simulink library "World_Config_Utilities"  (R2022a)
settings: Solver=VariableStepAuto  StartTime=0.0  StopTime=10.0  RelTol=1e-3
undefined symbols (not defined in the file or in its folder): acc_theta, accel_ramp_rate, hp_rc_wld_t, qt, time_vector, xyz_matrix
libraries: sm_lib x6, nesl_utility x5, simulink x1, Scene_Systems x1, $bdroot x1
Description:
  | Simscape Vehicle Templates Library
  | 
  | Copyright 2018-2024 The MathWorks, Inc.
settings Model: Creator=smiller  LastModifiedBy=smiller

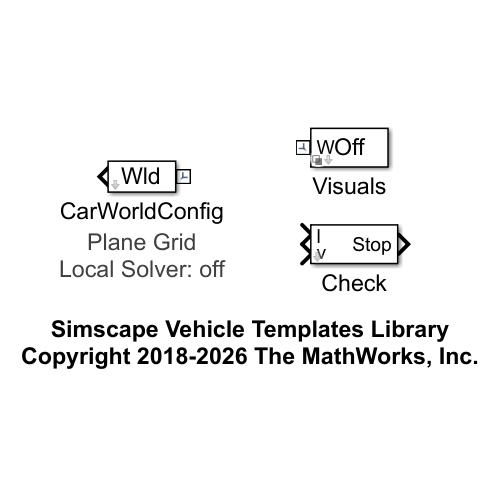
[thumbnail: Simulink's stored preview of the top-level diagram]
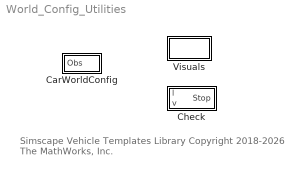
== system World_Config_Utilities ==
  note: Simscape Vehicle Templates Library
      | Copyright 2018-2026 The MathWorks, Inc.
  CarWorldConfig : Subsystem  mask(Environment){UseLocalSolver=off, LocalSolverChoice=Backward Euler, LocalSolverSampleTime=0.005, DoFixedCost=off, MaxNonlinIter=3, popup_scene=Plane Grid, popup_gravity=Constant, GravityVector=[0 0 -9.80665], popup_vis_point=Off, time_vector=qt, xyz_matrix=hp_rc_wld_t, clr_vis=[0.0 1.0 0.8], opc_vis=0.6, rad_vis=0.03}
      mask prompts: UseLocalSolver "Use Local Solver"; LocalSolverChoice "Solver Type:"; LocalSolverSampleTime "Sample time"; DoFixedCost "Use fixed-cost"; MaxNonlinIter "Number of iterations"; popup_scene "Scene"; popup_gravity "Gravity Model"; GravityVector "Gravity Vector [x y z] (m/s^2)"; popup_vis_point "Visualize Point"; time_vector "Time Vector [nx1] (sec)"; xyz_matrix "Coordinates [nx3] (m)"; clr_vis "Color [R G B] (0-1)"; opc_vis "Opacity (0-1)"; rad_vis "Radius (m)"
      mask help: World frame, driving surface, gravity, and solver settings.
      mask init:
      | if(LocalSolverChoice == 1)
      |     solverChoice = 'NE_BACKWARD_EULER_ADVANCER';
      | elseif(LocalSolverChoice == 2)
      |     solverChoice = 'NE_TRAPEZOIDAL_ADVANCER';
      | elseif(LocalSolverChoice == 3)
      |     solverChoice = 'NE_PARTITIONING_ADVANCER';
      | end
      | set_param([gcb '/Solver Configuration'],'LocalSolverChoice',solverChoice)
      | 
      | tempblkscenename = strrep(get_param(gcb,'popup_scene'),' ','_');
      | set_param([gcb '/Scene'],'LabelModeActiveChoice',tempblkscenename);
      | gravityModel = get_param(gcb,'popup_gravity');
      | if(strcmpi(gravityModel,'constant'))
      |     set_param([gcb '/Mechanism Configuration'],'LabelModeActiveChoice','ConstantGravity');
      | elseif(strcmpi(gravityModel,'ramp x and y components'))
      |     set_param([gcb '/Mechanism Configuration'],'LabelModeActiveChoice','VariableGravityXY');
      | end
      | clear tempblkscenename
      settings: AttributesFormatString=|
      | %<popup_scene>
      | Local Solver: %<UseLocalSolver>
      mask TypeOptions UseLocalSolver:
      | Solver
      | Configuration/UseLocalSolver
      mask Callback UseLocalSolver:
      | maskObj = Simulink.Mask.get(gcb);
      | 
      | samTM_h = maskObj.getParameter('LocalSolverSampleTime');
      | slvCH_h = maskObj.getParameter('LocalSolverChoice');
      | fixCT_h = maskObj.getParameter('DoFixedCost');
      | 
      | temp_useLSstate = get_param(gcb,'UseLocalSolver');
      | samTM_h.Enabled = temp_useLSstate;
      | slvCH_h.Enabled = temp_useLSstate;
      | fixCT_h.Enabled = temp_useLSstate;
      | 
      | clear maskObj
      | clear samTM_h slvCH_h fixCT_h
      | clear temp_useLSstate
      mask TypeOptions LocalSolverChoice: Backward Euler | Trapezoidal Rule | Partitioning
      mask TypeOptions LocalSolverSampleTime:
      | Solver
      | Configuration/LocalSolverSampleTime
      mask TypeOptions DoFixedCost:
      | Solver
      | Configuration/DoFixedCost
      mask Callback DoFixedCost:
      | maskObj = Simulink.Mask.get(gcb);
      | 
      | numIT_h = maskObj.getParameter('MaxNonlinIter');
      | 
      | temp_doFixCoststate = get_param(gcb,'DoFixedCost');
      | numIT_h.Enabled = temp_doFixCoststate;
      | 
      | clear maskObj numIT_h temp_doFixCoststate
      mask TypeOptions MaxNonlinIter:
      | Solver
      | Configuration/MaxNonlinIter
      mask TypeOptions popup_scene: Plane Grid | Road Two Lane | Double Lane Change | Double Lane Change ISO3888 | Slalom | Ice Patch | Elk Test | RDF Rough Road | Rough Road Z Only | CRG Rough Road | RDF Plateau | Plateau Z Only | CRG Plateau | Track Mallory Park | Track Mallory Park Obstacle | MCity | CRG Hockenheim | CRG Hockenheim F | CRG Kyalami | CRG Kyalami F | CRG Mallory Park | CRG Mallory Park F | CRG Nurburgring N | CRG Nurburgring N F | CRG Pikes Peak | CRG Suzuka | CRG Suzuka F | CRG Custom | CRG Custom F | GS Uneven Road | GS Grid Surface | Skidpad | Constant Radius | Testrig 4 Post
      mask TypeOptions popup_gravity: Constant | Ramp x and y components
      mask TypeOptions popup_vis_point: Visuals/popup_vis_point
      mask Callback popup_vis_point:
      | bh = gcb;
      | maskObj = Simulink.Mask.get(bh); % Get the mask object of the current block
      | tvec_h  = maskObj.getParameter('time_vector'); % Get the parameter to hide
      | xyz_h   = maskObj.getParameter('xyz_matrix'); % Get the parameter to hide
      | 
      | clr_h   = maskObj.getParameter('clr_vis'); % Get the parameter to hide
      | opc_h   = maskObj.getParameter('opc_vis'); % Get the parameter to hide
      | rad_h   = maskObj.getParameter('rad_vis'); % Get the parameter to hide
      | 
      | % Check the value of ControlParam
      | enaVisPnt = get_param(bh, 'popup_vis_point');
      | 
      | tvec_h.Visible  = 'off';
      | xyz_h.Visible  = 'off';
      | clr_h.Visible  = 'off';
      | opc_h.Visible  = 'off';
      | rad_h.Visible  = 'off';
      | 
      | if strcmp(enaVisPnt, 'On')
      |     tvec_h.Visible  = 'on';
      |     xyz_h.Visible   = 'on';
      |     clr_h.Visible   = 'on';
      |     opc_h.Visible   = 'on';
      |     rad_h.Visible   = 'on';
      | end
      mask TypeOptions time_vector: Visuals/time_vector
      mask TypeOptions xyz_matrix: Visuals/xyz_matrix
      mask TypeOptions clr_vis: Visuals/clr_vis
      mask TypeOptions opc_vis: Visuals/opc_vis
      mask TypeOptions rad_vis: Visuals/rad_vis
      mask Display: disp('Wld')
  Check : Subsystem  mask(Stop Conditions){stop_speed=0.1, start_check_time=5, max_speed=0.4, start_check_time_max_speed=20000, lat_dev_threshold=8, start_check_time_ld=10000, end_lap_num=1, start_check_time_end_lap=10000, max_dist_threshold=10000, start_check_time_max_dist=10000}
      mask help: Check conditions of vehicle to determine if simulation should stop. Conditions can include speed, position, or end of lap. Set time to start check to very high values to prevent condition from stopping simulation.
      mask TypeOptions stop_speed: Stop Threshold/Value
      mask TypeOptions start_check_time: Start Checking/Time
      mask TypeOptions max_speed: Max Speed Threshold/Value
      mask TypeOptions start_check_time_max_speed: Start Checking Max Speed/Time
      mask TypeOptions lat_dev_threshold: Lateral Deviation Threshold/Value
      mask TypeOptions start_check_time_ld: Start Checking Lat Dev/Time
      mask TypeOptions end_lap_num: End Lap/Value
      mask TypeOptions start_check_time_end_lap: Start Checking End Lap/Time
      mask TypeOptions max_dist_threshold: End Distance/Value
      mask TypeOptions start_check_time_max_dist: Start Checking End Distance/Time
      mask DialogControl text_quantity Prompt: Quantity
      mask DialogControl text_start_check Prompt: Start Check (sec)
      mask DialogControl text_final_speed Prompt: Final Speed (m/s)
      mask DialogControl text_max_speed Prompt: Max Speed (m/s)
      mask DialogControl text_max_lat_dev Prompt: Max Lateral Offset (m)
      mask DialogControl text_end_lap_1 Prompt: End Lap
      mask DialogControl text_max_distance Prompt: Max Distance
  Visuals : Subsystem  Variant=on  VariantControlMode=label  VariantControl=Choice  LabelModeActiveChoice=Off  mask{popup_vis_point=Off, time_vector=time_vector, xyz_matrix=xyz_matrix, clr_vis=[0.0 1.0 0.8], opc_vis=0.6, rad_vis=0.03}
      mask prompts: popup_vis_point "Visualize Point"; time_vector "Time Vector [nx1] (sec)"; xyz_matrix "Coordinates [nx3] (m)"; clr_vis "Color [R G B] (0-1)"; opc_vis "Opacity (0-1)"; rad_vis "Radius (m)"
      mask init:
      | bh = gcb;
      | pvisPt = get_param(bh,'popup_vis_point');
      | if(strcmp(pvisPt,'Off'))
      |     time_vector = [0];
      |     xyz_matrix =  [0 0 0];
      | end
      | set_param(bh,'LabelModeActiveChoice',pvisPt)
      mask TypeOptions popup_vis_point: Off | On
      mask Callback popup_vis_point:
      | bh = gcb;
      | maskObj = Simulink.Mask.get(bh); % Get the mask object of the current block
      | tvec_h  = maskObj.getParameter('time_vector'); % Get the parameter to hide
      | xyz_h   = maskObj.getParameter('xyz_matrix'); % Get the parameter to hide
      | clr_h   = maskObj.getParameter('clr_vis'); % Get the parameter to hide
      | opc_h   = maskObj.getParameter('opc_vis'); % Get the parameter to hide
      | rad_h   = maskObj.getParameter('rad_vis'); % Get the parameter to hide
      | 
      | % Check the value of ControlParam
      | enaVisPnt = get_param(bh, 'popup_vis_point');
      | 
      | tvec_h.Visible  = 'off';
      | xyz_h.Visible  = 'off';
      | clr_h.Visible  = 'off';
      | opc_h.Visible  = 'off';
      | rad_h.Visible  = 'off';
      | 
      | if strcmp(enaVisPnt, 'On')
      |     tvec_h.Visible  = 'on';
      |     xyz_h.Visible   = 'on';
      |     clr_h.Visible   = 'on';
      |     opc_h.Visible   = 'on';
      |     rad_h.Visible   = 'on';
      | end

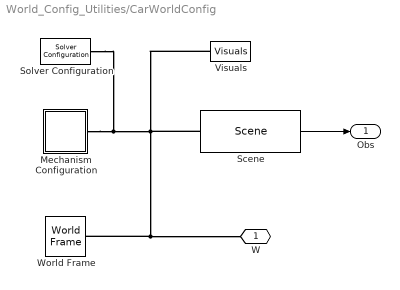
== system World_Config_Utilities/CarWorldConfig ==
  Mechanism Configuration : Subsystem  Variant=on  VariantControlMode=label  VariantControl=Choice  LabelModeActiveChoice=ConstantGravity
      settings: AttributesFormatString=%<LabelModeActiveChoice>
      mask Display: disp(' ');
  Scene : Scene_Systems/Scene  SystemSampleTime=-1  LabelModeActiveChoice=Plane_Grid  VariantActivationTime=update diagram  Latency=0  AutoFrameSizeCalculation=off
      settings: AttributesFormatString=%<LabelModeActiveChoice>
  Solver Configuration : nesl_utility/Solver Configuration  PhysicalDomain=network_engine_domain  SubClassName=solver  LeftPortType=input  RightPortType=generic  Tones=[]  Harmonics=[]  SimulateNoise=off  Profile=off  UseLocalSampling=off  EnableSwitchedLinearOptims=on  FrequencyDomain=off  UseCCode=off  RelTol=0.001  AbsTol=1e-06  MinStep=1e-09  ToWorkspace=off  RevertToSquareIcSolve=off  NumHomotopyIterations=100  PhasorMode=off  PhasorModeNumHarmonics=1  IndexReductionMethod=DerivativeReplacement  DoDC=off  ResidualTolerance=1e-9  UseLocalSolver=off  LocalSolverChoice=NE_BACKWARD_EULER_ADVANCER  LocalSolverSampleTime=LocalSolverSampleTime  DoFixedCost=off  MaxNonlinIter=MaxNonlinIter  MaxModeIter=2  ComputeImpulses=off  ImpulseIterations=2  LinearAlgebra=Sparse  LinearAlgebraNumThread=0  EquationFormulation=NE_TIME_EF  DelaysMemoryBudget=1024  AutomaticFiltering=on  FilteringTimeConstant=0.001  PartitionStorageMethod=AS_NEEDED  PartitionMemoryBudget=1024  PartitionMethod=FAST
      settings: SourceProductBaseCode=SS,PW,VE
  Visuals : $bdroot/Visuals  VariantControl=Choice  LabelModeActiveChoice=Off  popup_vis_point=Off  time_vector=time_vector  xyz_matrix=xyz_matrix  clr_vis=clr_vis  opc_vis=opc_vis  rad_vis=rad_vis
  World Frame : sm_lib/Frames and Transforms/World Frame
  W : PMIOPort  Side=Left
  Obs : Outport  VectorParamsAs1DForOutWhenUnconnected=off
  wires:
  Scene/1 -> Obs/1
  connections:
  Solver Configuration/RConn1 -- Mechanism Configuration/RConn1 -- Visuals/LConn1 -- World Frame/RConn1 -- W/RConn1 -- Scene/LConn1

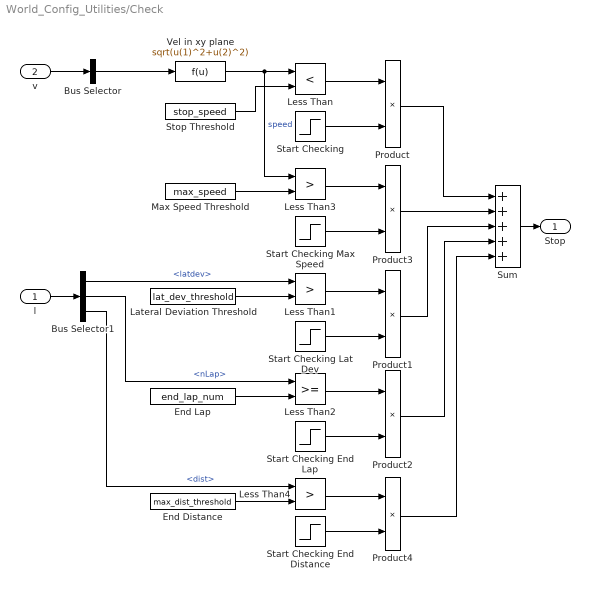
== system World_Config_Utilities/Check ==
  l : Inport
  v : Inport  Port=2
  Bus Selector : BusSelector  OutputSignals=World.vx,World.vy  OutputAsBus=on
  Bus Selector1 : BusSelector  OutputSignals=Reference.latdev,Reference.nLap,Reference.dist
  End Distance : Constant  Value=max_dist_threshold
  End Lap : Constant  Value=end_lap_num
  Lateral Deviation Threshold : Constant  Value=lat_dev_threshold
  Less Than : RelationalOperator  Operator=<  OutDataTypeStr=boolean  RndMeth=Simplest  InputSameDT=off
  Less Than1 : RelationalOperator  Operator=>  OutDataTypeStr=boolean  ZeroCross=off  RndMeth=Simplest  InputSameDT=off
  Less Than2 : RelationalOperator  OutDataTypeStr=boolean  RndMeth=Simplest  InputSameDT=off
  Less Than3 : RelationalOperator  Operator=>  OutDataTypeStr=boolean  RndMeth=Simplest  InputSameDT=off
  Less Than4 : RelationalOperator  Operator=>  OutDataTypeStr=boolean  ZeroCross=off  RndMeth=Simplest  InputSameDT=off
  Max Speed Threshold : Constant  Value=max_speed
  Product{,1..4} (5 alike) : Product
  Start Checking : Step  Time=start_check_time  SampleTime=0  ZeroCross=off
  Start Checking End Distance : Step  Time=start_check_time_max_dist  SampleTime=0  ZeroCross=off
  Start Checking End Lap : Step  Time=start_check_time_end_lap  SampleTime=0  ZeroCross=off
  Start Checking Lat Dev : Step  Time=start_check_time_ld  SampleTime=0  ZeroCross=off
  Start Checking Max Speed : Step  Time=start_check_time_max_speed  SampleTime=0  ZeroCross=off
  Stop Threshold : Constant  Value=stop_speed
  Sum : Sum  Inputs=+++++
  Vel in xy plane : Fcn  Expr=sqrt(u(1)^2+u(2)^2)
  Stop : Outport  VectorParamsAs1DForOutWhenUnconnected=off
  wires:
  Bus Selector1/2 -> Less Than2/1  "<nLap>"
  Product3/1 -> Sum/2
  Max Speed Threshold/1 -> Less Than3/2
  Less Than3/1 -> Product3/1
  Start Checking Max Speed/1 -> Product3/2
  Product2/1 -> Sum/4
  Start Checking End Lap/1 -> Product2/2
  Less Than2/1 -> Product2/1
  End Lap/1 -> Less Than2/2
  Product1/1 -> Sum/3
  Sum/1 -> Stop/1
  Start Checking Lat Dev/1 -> Product1/2
  Less Than1/1 -> Product1/1
  Lateral Deviation Threshold/1 -> Less Than1/2
  Bus Selector1/1 -> Less Than1/1  "<latdev>"
  l/1 -> Bus Selector1/1
  Vel in xy plane/1 -> Less Than3/1, Less Than/1  "speed"
  Bus Selector/1 -> Vel in xy plane/1
  Product/1 -> Sum/1
  Start Checking/1 -> Product/2
  v/1 -> Bus Selector/1
  Stop Threshold/1 -> Less Than/2
  Less Than/1 -> Product/1
  End Distance/1 -> Less Than4/2
  Bus Selector1/3 -> Less Than4/1  "<dist>"
  Less Than4/1 -> Product4/1
  Start Checking End Distance/1 -> Product4/2
  Product4/1 -> Sum/5

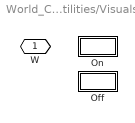
== system World_Config_Utilities/Visuals ==
  Off : Subsystem  VariantControl=Off
  On : Subsystem  VariantControl=On  mask{tvec=time_vector, visp1=xyz_matrix, clr_vis=clr_vis, opc_vis=opc_vis, rad_vis=rad_vis}
      mask prompts: tvec "Time Vector (s)"; visp1 "Coordinates [x y z] (s)"; clr_vis "Color [R G B] (0-1)"; opc_vis "Opacity (0-1)"; rad_vis "Radius (m)"
      mask init:
      | % Ensure matrices have correct dimensions
      | if(size(tvec,2)>1)
      |     t_vec = tvec';
      | else
      |     t_vec = tvec;
      | end
      | 
      | if(size(visp1,2)>3)
      |     vis_p1 = visp1';
      | else
      |     vis_p1 = visp1;
      | end
      | 
      | if((size(t_vec,1)==size(vis_p1,1)) && ...
      |         size(vis_p1,2)==3)
      | else
      |     % If not valid set of data, leave vis at [0 0 0]
      |     % and warn user.
      |     t_vec = 0;
      |     vis_p1 = [0 0 0];
      |     warning('Visualization data not defined correctly.')
      | end
  W : PMIOPort  Side=Left

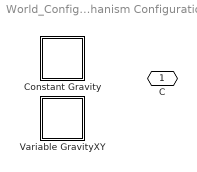
== system World_Config_Utilities/CarWorldConfig/Mechanism Configuration ==
  Constant Gravity : Subsystem  VariantControl=ConstantGravity
  Variable GravityXY : Subsystem  VariantControl=VariableGravityXY
  C : PMIOPort  Side=Right

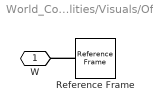
== system World_Config_Utilities/Visuals/Off ==
  Reference Frame : sm_lib/Frames and Transforms/Reference Frame
  W : PMIOPort  Side=Left
  connections:
  Reference Frame/RConn1 -- W/RConn1

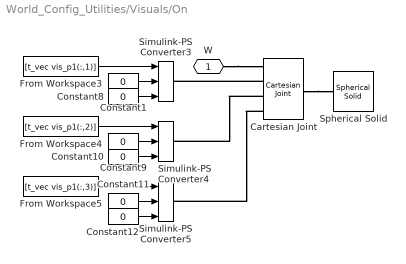
== system World_Config_Utilities/Visuals/On ==
  Cartesian Joint : sm_lib/Joints/Cartesian Joint  JointMode=Normal  SenseConstraintForce=off  SenseConstraintForceX=off  SenseConstraintForceY=off  SenseConstraintForceZ=off  SenseConstraintTorque=off  SenseConstraintTorqueX=off  SenseConstraintTorqueY=off  SenseConstraintTorqueZ=off  SenseTotalForce=off  SenseTotalForceX=off  SenseTotalForceY=off  SenseTotalForceZ=off  SenseTotalTorque=off  SenseTotalTorqueX=off  SenseTotalTorqueY=off  SenseTotalTorqueZ=off  CompositeWrenchDir=FollowerOnBase  CompositeWrenchFrame=BaseFrame  PxEquilibriumPosition=0  PxEquilibriumPositionUnits=m  PxSpringStiffness=0  PxSpringStiffnessUnits=N/m  PxDampingCoefficient=0  PxDampingCoefficientUnits=N/(m/s)  PxTorqueActuationMode=ComputedTorque  PxMotionActuationMode=InputMotion  PxSensePosition=off  PxSenseVelocity=off  PxSenseAcceleration=off  PxSenseTorqueForce=off  PxSenseLowerLimitTorqueForce=off  PxSenseUpperLimitTorqueForce=off  PxLowerLimitSpecify=off  PxLowerLimitBound=-1  PxLowerLimitBoundUnits=m  PxLowerLimitStiffness=1e6  PxLowerLimitStiffnessUnits=N/m  PxLowerLimitDamping=1e3  PxLowerLimitDampingUnits=N/(m/s)  PxLowerLimitTransitionRegionWidth=1e-4  PxLowerLimitTransitionRegionWidthUnits=m  PxUpperLimitSpecify=off  PxUpperLimitBound=1  PxUpperLimitBoundUnits=m  PxUpperLimitStiffness=1e6  PxUpperLimitStiffnessUnits=N/m  PxUpperLimitDamping=1e3  PxUpperLimitDampingUnits=N/(m/s)  PxUpperLimitTransitionRegionWidth=1e-4  PxUpperLimitTransitionRegionWidthUnits=m  PxPositionTargetSpecify=off  PxPositionTargetPriority=High  PxPositionTargetValue=0  PxPositionTargetValueUnits=m  PxVelocityTargetSpecify=off  PxVelocityTargetPriority=High  PxVelocityTargetValue=0  PxVelocityTargetValueUnits=m/s  PyEquilibriumPosition=0  PyEquilibriumPositionUnits=m  PySpringStiffness=0  PySpringStiffnessUnits=N/m  PyDampingCoefficient=0  PyDampingCoefficientUnits=N/(m/s)  PyTorqueActuationMode=ComputedTorque  PyMotionActuationMode=InputMotion  PySensePosition=off  PySenseVelocity=off  PySenseAcceleration=off  PySenseTorqueForce=off  PySenseLowerLimitTorqueForce=off  PySenseUpperLimitTorqueForce=off  PyLowerLimitSpecify=off  PyLowerLimitBound=-1  PyLowerLimitBoundUnits=m  PyLowerLimitStiffness=1e6  PyLowerLimitStiffnessUnits=N/m  PyLowerLimitDamping=1e3  PyLowerLimitDampingUnits=N/(m/s)  PyLowerLimitTransitionRegionWidth=1e-4  PyLowerLimitTransitionRegionWidthUnits=m  PyUpperLimitSpecify=off  PyUpperLimitBound=1  PyUpperLimitBoundUnits=m  PyUpperLimitStiffness=1e6  PyUpperLimitStiffnessUnits=N/m  PyUpperLimitDamping=1e3  PyUpperLimitDampingUnits=N/(m/s)  PyUpperLimitTransitionRegionWidth=1e-4  PyUpperLimitTransitionRegionWidthUnits=m  PyPositionTargetSpecify=off  PyPositionTargetPriority=High  PyPositionTargetValue=0  PyPositionTargetValueUnits=m  PyVelocityTargetSpecify=off  PyVelocityTargetPriority=High  PyVelocityTargetValue=0  PyVelocityTargetValueUnits=m/s  PzEquilibriumPosition=0  PzEquilibriumPositionUnits=m  PzSpringStiffness=0  PzSpringStiffnessUnits=N/m  PzDampingCoefficient=0  PzDampingCoefficientUnits=N/(m/s)  PzTorqueActuationMode=ComputedTorque  PzMotionActuationMode=InputMotion  PzSensePosition=off  PzSenseVelocity=off  PzSenseAcceleration=off  PzSenseTorqueForce=off  PzSenseLowerLimitTorqueForce=off  PzSenseUpperLimitTorqueForce=off  PzLowerLimitSpecify=off  PzLowerLimitBound=-1  PzLowerLimitBoundUnits=m  PzLowerLimitStiffness=1e6  PzLowerLimitStiffnessUnits=N/m  PzLowerLimitDamping=1e3  PzLowerLimitDampingUnits=N/(m/s)  PzLowerLimitTransitionRegionWidth=1e-4  PzLowerLimitTransitionRegionWidthUnits=m  PzUpperLimitSpecify=off  PzUpperLimitBound=1  PzUpperLimitBoundUnits=m  PzUpperLimitStiffness=1e6  PzUpperLimitStiffnessUnits=N/m  PzUpperLimitDamping=1e3  PzUpperLimitDampingUnits=N/(m/s)  PzUpperLimitTransitionRegionWidth=1e-4  PzUpperLimitTransitionRegionWidthUnits=m  PzPositionTargetSpecify=off  PzPositionTargetPriority=High  PzPositionTargetValue=0  PzPositionTargetValueUnits=m  PzVelocityTargetSpecify=off  PzVelocityTargetPriority=High  PzVelocityTargetValue=0  PzVelocityTargetValueUnits=m/s
  Constant{1,8..12} (6 alike) : Constant  Value=0
  From Workspace3 : FromWorkspace  VariableName=[t_vec vis_p1(:,1)]
  From Workspace4 : FromWorkspace  VariableName=[t_vec vis_p1(:,2)]
  From Workspace5 : FromWorkspace  VariableName=[t_vec vis_p1(:,3)]
  Simulink-PS Converter3 : nesl_utility/Simulink-PS Converter  PhysicalDomain=network_engine_domain  SubClassName=ps_input  LeftPortType=input  RightPortType=output  PseudoPeriodic=off  Frequencies=[]  NoiseDistribution=none  NoiseParameters=[]  Unit=1  AffineConversion=off  FilteringAndDerivatives=provide  SimscapeFilterOrder=1  InputFilterTimeConstant=0.001  UdotUserProvided=2
      settings: SourceProductBaseCode=SS,PW,VE
  Simulink-PS Converter4 : nesl_utility/Simulink-PS Converter  PhysicalDomain=network_engine_domain  SubClassName=ps_input  LeftPortType=input  RightPortType=output  PseudoPeriodic=off  Frequencies=[]  NoiseDistribution=none  NoiseParameters=[]  Unit=1  AffineConversion=off  FilteringAndDerivatives=provide  SimscapeFilterOrder=1  InputFilterTimeConstant=0.001  UdotUserProvided=2
      settings: SourceProductBaseCode=SS,PW,VE
  Simulink-PS Converter5 : nesl_utility/Simulink-PS Converter  PhysicalDomain=network_engine_domain  SubClassName=ps_input  LeftPortType=input  RightPortType=output  PseudoPeriodic=off  Frequencies=[]  NoiseDistribution=none  NoiseParameters=[]  Unit=1  AffineConversion=off  FilteringAndDerivatives=provide  SimscapeFilterOrder=1  InputFilterTimeConstant=0.001  UdotUserProvided=2
      settings: SourceProductBaseCode=SS,PW,VE
  Spherical Solid : sm_lib/Body Elements/Spherical Solid  GraphicAmbientColor=[0.15 0.15 0.15 1.0]  BasedOnType=Mass  CenterOfMass=[0 0 0]  CenterOfMassUnits=m  GraphicDiffuseColor=clr_vis  Density=1000  DensityUnits=kg/m^3  DoExposeReferenceFrame=on  GraphicEmissiveColor=[0.0 0.0 0.0 1.0]  ExportEntireGeometry=off  SerializedExposedGeometries=<ExposedGeometries/>  SerializedFrames=<Frames/>  MarkerShape=Sphere  MarkerSize=10  GraphicType=FromGeometry  InertiaType=CalculateFromGeometry  Mass=1e-3  MassUnits=kg  MomentsOfInertia=[1 1 1]  MomentsOfInertiaUnits=kg*m^2  GraphicOpacity=opc_vis  ProductsOfInertia=[0 0 0]  ProductsOfInertiaUnits=kg*m^2  GraphicShininess=75  GraphicSpecularColor=[0.5 0.5 0.5 1.0]  SphereRadius=rad_vis  SphereRadiusUnits=m  GraphicVisPropType=SimpleVisualProperties
  W : PMIOPort  Side=Left
  wires:
  Constant12/1 -> Simulink-PS Converter5/3
  Constant11/1 -> Simulink-PS Converter5/2
  From Workspace5/1 -> Simulink-PS Converter5/1
  From Workspace3/1 -> Simulink-PS Converter3/1
  Constant9/1 -> Simulink-PS Converter4/2
  Constant10/1 -> Simulink-PS Converter4/3
  Constant1/1 -> Simulink-PS Converter3/2
  Constant8/1 -> Simulink-PS Converter3/3
  From Workspace4/1 -> Simulink-PS Converter4/1
  connections:
  W/RConn1 -- Cartesian Joint/LConn1
  Cartesian Joint/RConn1 -- Spherical Solid/RConn1
  Cartesian Joint/LConn4 -- Simulink-PS Converter5/RConn1
  Cartesian Joint/LConn3 -- Simulink-PS Converter4/RConn1
  Cartesian Joint/LConn2 -- Simulink-PS Converter3/RConn1

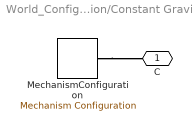
== system World_Config_Utilities/CarWorldConfig/Mechanism Configuration/Constant Gravity ==
  MechanismConfiguration : sm_lib/Utilities/Mechanism Configuration  UniformGravity=Constant  GravityVector=GravityVector  GravityUnits=m/s^2  LinearizationDelta=0.001  JointModeTransitionNonlinearIterations=2
  C : PMIOPort  Side=Right
  connections:
  MechanismConfiguration/RConn1 -- C/RConn1

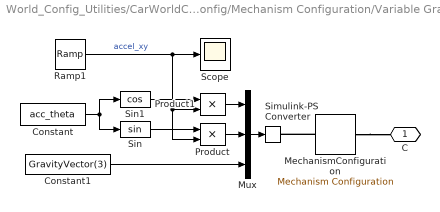
== system World_Config_Utilities/CarWorldConfig/Mechanism Configuration/Variable GravityXY ==
  Constant : Constant  Value=acc_theta
  Constant1 : Constant  Value=GravityVector(3)
  MechanismConfiguration : sm_lib/Utilities/Mechanism Configuration  UniformGravity=TimeVarying  GravityVector=[0 0 -9.80665]  GravityUnits=m/s^2  LinearizationDelta=0.001  JointModeTransitionNonlinearIterations=2
  Mux : Mux  Inputs=3
  Product : Product
  Product1 : Product
  Ramp1 : simulink/Sources/Ramp  slope=accel_ramp_rate  start=2  InitialOutput=0
  Scope : Scope
  Simulink-PS Converter : nesl_utility/Simulink-PS Converter  PhysicalDomain=network_engine_domain  SubClassName=ps_input  LeftPortType=input  RightPortType=output  PseudoPeriodic=off  Frequencies=[]  NoiseDistribution=none  NoiseParameters=[]  Unit=m/s^2  AffineConversion=off  FilteringAndDerivatives=provide  SimscapeFilterOrder=1  InputFilterTimeConstant=0.001  UdotUserProvided=0
      settings: SourceProductBaseCode=SS,PW,VE
  Sin : Trigonometry
  Sin1 : Trigonometry  Operator=cos
  C : PMIOPort  Side=Right
  wires:
  Product/1 -> Mux/2
  Constant/1 -> Sin1/1, Sin/1
  Sin1/1 -> Product1/1
  Mux/1 -> Simulink-PS Converter/1
  Sin/1 -> Product/1
  Constant1/1 -> Mux/3
  Product1/1 -> Mux/1
  Ramp1/1 -> Scope/1, Product1/2, Product/2  "accel_xy"
  connections:
  MechanismConfiguration/RConn1 -- C/RConn1
  MechanismConfiguration/LConn1 -- Simulink-PS Converter/RConn1
